simulink model "orbit_propogator_kep"  (R2023b)
settings: Solver=FixedStepAuto  StartTime=0  StopTime=5929*3  FixedStep=50  RelTol=1e-3
settings Model: Creator=annahylbert  LastModifiedBy=annahylbert

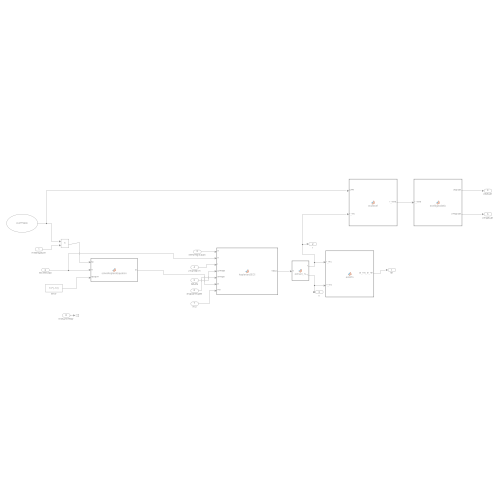
[thumbnail: Simulink's stored preview of the top-level diagram]
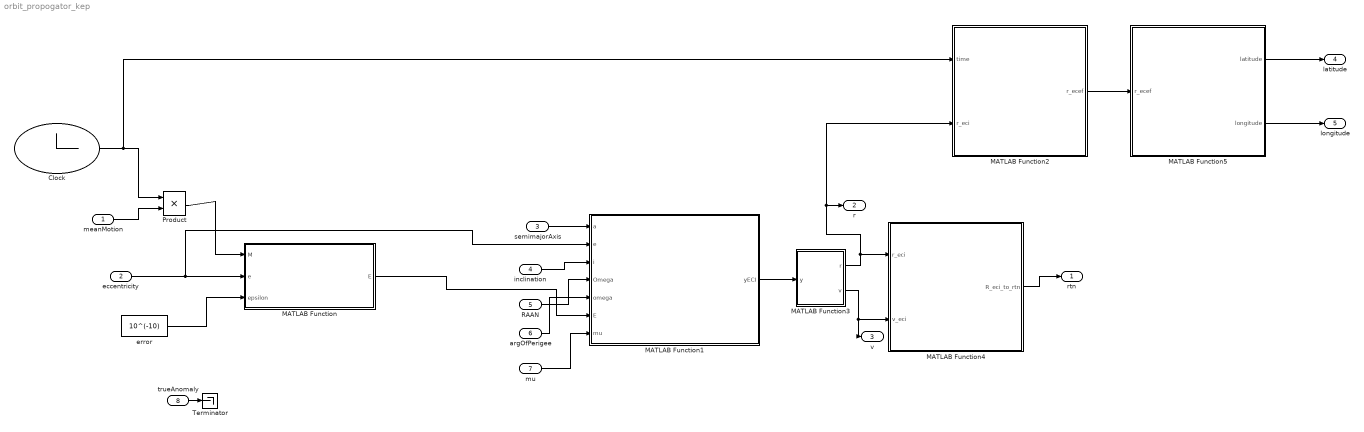
== system orbit_propogator_kep ==
  meanMotion : Inport
  eccentricity : Inport  Port=2
  semimajorAxis : Inport  Port=3
  inclination : Inport  Port=4
  RAAN : Inport  Port=5
  argOfPerigee : Inport  Port=6
  mu : Inport  Port=7
  trueAnomaly : Inport  Port=8
  Clock : Clock
      settings: Decimation=99999999
  MATLAB Function : MATLAB Function  TreatAsAtomicUnit=on
  MATLAB Function1 : MATLAB Function  TreatAsAtomicUnit=on
  MATLAB Function2 : MATLAB Function  TreatAsAtomicUnit=on
  MATLAB Function3 : MATLAB Function  TreatAsAtomicUnit=on
  MATLAB Function4 : MATLAB Function  TreatAsAtomicUnit=on
  MATLAB Function5 : MATLAB Function  TreatAsAtomicUnit=on
  Product : Product
  Terminator : Terminator
  error : Constant  Value=10^(-10)
  rtn : Outport
  r : Outport  Port=2
  v : Outport  Port=3
  latitude : Outport  Port=4
  longitude : Outport  Port=5
  wires:
  eccentricity/1 -> MATLAB Function1/2(e), MATLAB Function/2(e)
  Product/1 -> MATLAB Function/1(M)
  meanMotion/1 -> Product/2
  error/1 -> MATLAB Function/3(epsilon)
  MATLAB Function/1(E) -> MATLAB Function1/6(E)
  semimajorAxis/1 -> MATLAB Function1/1(a)
  inclination/1 -> MATLAB Function1/3(i)
  RAAN/1 -> MATLAB Function1/4(Omega)
  argOfPerigee/1 -> MATLAB Function1/5(omega)
  MATLAB Function3/2(v) -> v/1, MATLAB Function4/2(v_eci)
  MATLAB Function4/1(R_eci_to_rtn) -> rtn/1
  MATLAB Function1/1(yECI) -> MATLAB Function3/1(y)
  MATLAB Function3/1(r) -> MATLAB Function2/2(r_eci), r/1, MATLAB Function4/1(r_eci)
  MATLAB Function2/1(r_ecef) -> MATLAB Function5/1(r_ecef)
  Clock/1 -> MATLAB Function2/1(time), Product/1
  MATLAB Function5/1(latitude) -> latitude/1
  MATLAB Function5/2(longitude) -> longitude/1
  mu/1 -> MATLAB Function1/7(mu)
  trueAnomaly/1 -> Terminator/1

== matlab function orbit_propogator_kep/MATLAB Function1 ==
  data: a input; yECI output; e input; i input; Omega input; omega input; E input; mu input
function yECI   = keplerian2ECI(a, e, i, Omega, omega, E, mu)

    % Calculate position and velocity in the perifocal coordinate system
    n = sqrt(mu/a^3);
    r_perifocal = [a*(cos(E) - e); a*sin(E)*sqrt(1-e^2); 0];
    v_perifocal = a*n/(1-e*cos(E)) * [-sin(E); cos(E)*sqrt(1-e^2); 0];

    % Rotation matrices
    R3_Omega = [cos(-Omega) sin(-Omega) 0;
                -sin(-Omega) cos(-Omega) 0;
                0 0 1];
    R1_i = [1 0 0;
            0 cos(-i) sin(-i);
            0 -sin(-i) cos(-i)];
    R3_omega = [cos(-omega) sin(-omega) 0;
                -sin(-omega) cos(-omega) 0;
                0 0 1];

    % Transformation to ECI
    Q_perifocal2ECI = R3_Omega * R1_i * R3_omega;
    rECI = Q_perifocal2ECI * r_perifocal;
    vECI = Q_perifocal2ECI * v_perifocal;

    yECI = [rECI; vECI];
end

== matlab function orbit_propogator_kep/MATLAB Function ==
  data: M input; E output; e input; epsilon input
function E = solveKeplersEquation(M, e, epsilon)
    E = M; % Initial Guess
    while true
        E_new = E - (E - e*sin(E) - M) / (1 - e*cos(E)); % Newton-Raphson iteration
        if abs(E_new - E) < epsilon
            break; % Convergence reached
        end
        E = E_new;
    end
end

== matlab function orbit_propogator_kep/MATLAB Function3 ==
  data: r output; y input; v output
function [r,v] = extract_rv(y)
    % Define the equations of motion for orbital derivatives
    r = y(1:3);
    v = y(4:6);
end

== matlab function orbit_propogator_kep/MATLAB Function4 ==
  data: R_eci_to_rtn output; r_eci input; v_eci input
function R_eci_to_rtn = eci2rtn(r_eci, v_eci)
    
    % Compute radial, transverse, and normal vectors in ECI frame
    r_radial_eci = r_eci;
    r_normal_eci = cross(r_radial_eci, v_eci);
    r_transverse_eci = -cross(r_radial_eci, r_normal_eci);
    
    % Normalize radial, transverse, and normal vectors to obtain unit vectors
    r_radial_eci_unit = r_radial_eci / norm(r_radial_eci);
    r_transverse_eci_unit = r_transverse_eci / norm(r_transverse_eci);
    r_normal_eci_unit = r_normal_eci / norm(r_normal_eci);
    
    % Construct rotation matrix from ECI to RTN
    R_eci_to_rtn = [r_radial_eci_unit, r_transverse_eci_unit, r_normal_eci_unit];

end

== matlab function orbit_propogator_kep/MATLAB Function2 ==
  data: r_ecef output; time input; r_eci input
function r_ecef   = eci2ecef(time, r_eci)

    D = time/(24*60*60);

    mjd = 59987.6458 + D;

    d = mjd - 51544.5;
    gmst_deg = 280.4606 + (360.9856473*d);
    gmst_rad = deg2rad(gmst_deg);

    % Step 1: Create rotation matrix for Earth's rotation about its axis
    R_z = [cos(gmst_rad), -sin(gmst_rad), 0;
           sin(gmst_rad), cos(gmst_rad),  0;
           0,               0,               1];

    % Step 2: Transpose the rotation matrix
    R = transpose(R_z);

    r_ecef = R*r_eci;

end

== matlab function orbit_propogator_kep/MATLAB Function5 ==
  data: latitude output; r_ecef input; longitude output
function [latitude, longitude] = ecef2geodetic(r_ecef)
    % go from ecef to geocentric 
    rx = r_ecef(1);
    ry = r_ecef(2);
    rz = r_ecef(3);

    longitude = atan2(ry, rx);
    latitude = atan2(rz, sqrt(rx^2 + ry^2));
end
